simulink model "Andrej_Klein_zadanie2B"  (R2022b)
settings: Solver=VariableStepAuto  StartTime=0.0  StopTime=30  RelTol=1e-3
model workspace (MAT data in the model file):
  FSX1 : sugfis (value not decoded)
  FSX2 : sugfis (value not decoded)
  Sig = Simulink.Signal
  Sig.DataType = 'auto'
  Sig.Dimensions = -1
  Sig.DimensionsMode = 'auto'
  Sig.Complexity = 'auto'
  Sig.SampleTime = -1
  Sig.SamplingMode = 'auto'
  T = 0.1
  a0 = 14.3
  a1 = 10
  a2 = 28
  b1 = 13
libraries: fuzblock x2, simulink x1
settings Model: Creator=hwswi  LastModifiedBy=hwswi
settings DataIOCC: ReturnWorkspaceOutputs=off

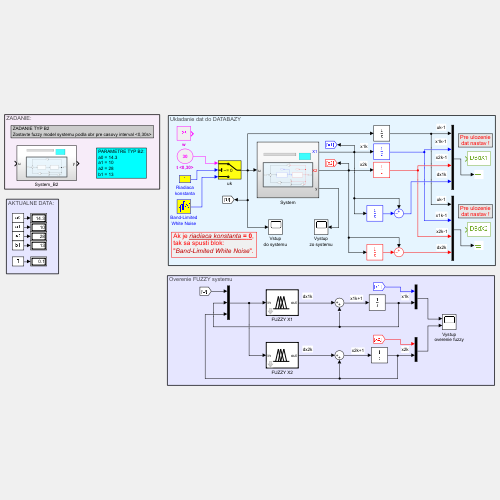
[thumbnail: Simulink's stored preview of the top-level diagram]
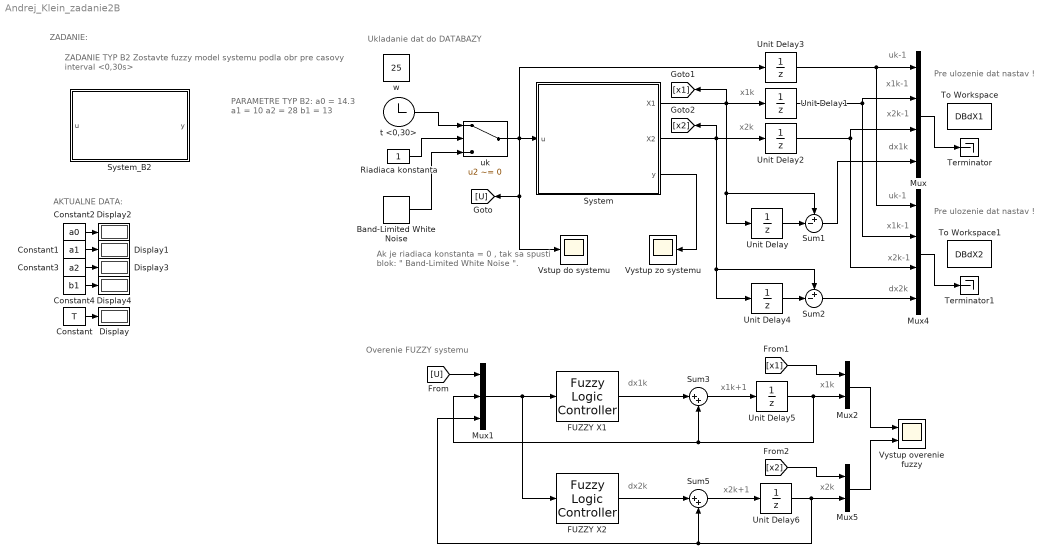
== system Andrej_Klein_zadanie2B ==
  note: Pre ulozenie
      | dat nastav !
  note: Ak je riadiaca konstanta = 0 ,
      | tak sa spusti blok:
      | " Band-Limited White Noise ".
  note: dx2k
  note: x1k+1
  note: x1k
  note: x1k
  note: uk-1
  note: Overenie FUZZY systemu
  note: AKTUALNE DATA:
  note: ZADANIE:
  note: Ukladanie dat do DATABAZY
  note: ZADANIE TYP B2
      | Zostavte fuzzy model systemu podla obr pre casovy interval <0,30s>
  note: PARAMETRE TYP B2:
      | a0 = 14.3
      | a1 = 10
      | a2 = 28
      | b1 = 13
  note: x1k-1
  note: dx1k
  note: x2k-1
  note: dx2k
  note: x2k
  note: x2k
  note: x2k+1
  note: dx1k
  note: uk-1
  note: x1k-1
  note: x2k-1
  note: Pre ulozenie
      | dat nastav !
  Band-Limited White Noise : simulink/Sources/Band-Limited White Noise  Cov=[500]  Ts=0.1  seed=[23341]
  Constant : Constant  Value=T
  Constant1 : Constant  Value=a1
  Constant2 : Constant  Value=a0
  Constant3 : Constant  Value=a2
  Constant4 : Constant  Value=b1
  Display{,1..4} (5 alike) : Display
  FUZZY X1 : fuzblock/Fuzzy Logic  Controller  FIS=FSX1  OutputSampleNumber=101  DataType=double  FuzzifiedInputs=off  RuleFiringStrengths=off  RuleOutputs=off  AggregatedOutputs=off  SimulateUsing=Interpreted execution  OutOfRangeInputValueMessage=warning  NoRuleFiredMessage=warning  EmptyOutputFuzzySetMessage=warning
  FUZZY X2 : fuzblock/Fuzzy Logic  Controller  FIS=FSX2  OutputSampleNumber=101  DataType=double  FuzzifiedInputs=off  RuleFiringStrengths=off  RuleOutputs=off  AggregatedOutputs=off  SimulateUsing=Interpreted execution  OutOfRangeInputValueMessage=warning  NoRuleFiredMessage=warning  EmptyOutputFuzzySetMessage=warning
  Mux : Mux
  Mux1 : Mux  Inputs=3
  Mux2 : Mux  Inputs=2
  Mux4 : Mux
  Mux5 : Mux  Inputs=2
  Riadiaca konstanta : Constant
  Sum1 : Sum  Inputs=+-|
  Sum2 : Sum  Inputs=+-|
  Sum3 : Sum  Inputs=|++
  Sum5 : Sum  Inputs=|++
  System : Subsystem
  System_B2 : Subsystem
  Terminator : Terminator
  Terminator1 : Terminator
  To Workspace : ToWorkspace  VariableName=DBdX1  SampleTime=0.1
  To Workspace1 : ToWorkspace  VariableName=DBdX2  SampleTime=0.1
  Unit Delay{,1..6} (7 alike) : UnitDelay  SampleTime=T
  Vstup do systemu : Scope
  Vystup overenie fuzzy : Scope  NumInputPorts=2
  Vystup zo systemu : Scope
  t <0,30> : Clock
  uk : Switch  Criteria=u2 ~= 0  Threshold=3  SaturateOnIntegerOverflow=off  InputSameDT=off
  w : Constant  Value=25
  wires:
  Constant/1 -> Display/1
  Constant1/1 -> Display1/1
  Constant2/1 -> Display2/1
  Constant3/1 -> Display3/1
  Constant4/1 -> Display4/1
  System/1(X1) -> [x1], Unit Delay1/1, Unit Delay/1, Sum1/1
  Unit Delay/1 -> Sum1/2
  Unit Delay4/1 -> Sum2/2
  System/2(X2) -> Unit Delay2/1, Sum2/1, Unit Delay4/1, [x2]
  Sum1/1 -> Mux/4
  Sum2/1 -> Mux4/4
  Unit Delay1/1 -> Mux/2, Mux4/2
  Unit Delay2/1 -> Mux4/3, Mux/3
  Unit Delay3/1 -> Mux/1, Mux4/1
  Sum3/1 -> Unit Delay5/1
  Unit Delay5/1 -> Sum3/2, Mux1/2, Mux2/2
  FUZZY X2/1 -> Sum5/1
  Unit Delay6/1 -> Mux5/2, Sum5/2, Mux1/3
  Sum5/1 -> Unit Delay6/1
  FUZZY X1/1 -> Sum3/1
  Mux5/1 -> Vystup overenie fuzzy/2
  Mux2/1 -> Vystup overenie fuzzy/1
  Mux1/1 -> FUZZY X2/1, FUZZY X1/1
  uk/1 -> System/1(u), [U], Vstup do systemu/1, Unit Delay3/1
  Riadiaca konstanta/1 -> uk/2
  Band-Limited White Noise/1 -> uk/3
  Mux/1 -> Terminator/1
  Mux4/1 -> Terminator1/1
  System/3(y) -> Vystup zo systemu/1
  [U] -> Mux1/1
  [x1] -> Mux2/1
  [x2] -> Mux5/1
  t <0,30>/1 -> uk/1

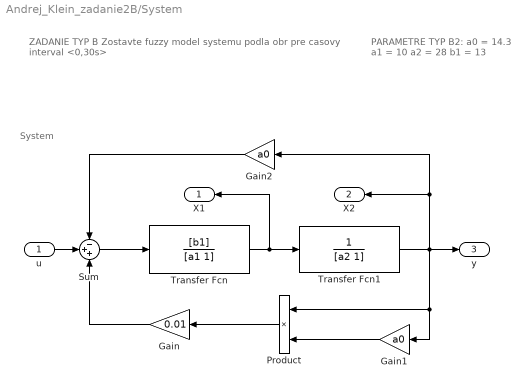
== system Andrej_Klein_zadanie2B/System ==
  note: System
  note: PARAMETRE TYP B2:
      | a0 = 14.3
      | a1 = 10
      | a2 = 28
      | b1 = 13
  note: ZADANIE TYP B
      | Zostavte fuzzy model systemu podla obr pre casovy interval <0,30s>
  u : Inport
  Gain : Gain  Gain=0.01
  Gain1 : Gain  Gain=a0
  Gain2 : Gain  Gain=a0
  Product : Product
  Sum : Sum  Inputs=-++
  Transfer Fcn : TransferFcn  Numerator=[b1]  Denominator=[a1 1]
  Transfer Fcn1 : TransferFcn  Denominator=[a2 1]
  X1 : Outport
  X2 : Outport  Port=2
  y : Outport  Port=3
  wires:
  Transfer Fcn/1 -> X1/1, Transfer Fcn1/1
  Transfer Fcn1/1 -> y/1, Gain2/1, X2/1, Gain1/1, Product/1
  Product/1 -> Gain/1
  Gain1/1 -> Product/2
  u/1 -> Sum/2
  Gain2/1 -> Sum/1
  Sum/1 -> Transfer Fcn/1
  Gain/1 -> Sum/3

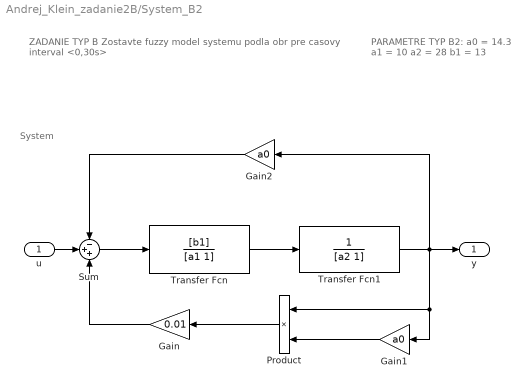
== system Andrej_Klein_zadanie2B/System_B2 ==
  note: System
  note: PARAMETRE TYP B2:
      | a0 = 14.3
      | a1 = 10
      | a2 = 28
      | b1 = 13
  note: ZADANIE TYP B
      | Zostavte fuzzy model systemu podla obr pre casovy interval <0,30s>
  u : Inport
  Gain : Gain  Gain=0.01
  Gain1 : Gain  Gain=a0
  Gain2 : Gain  Gain=a0
  Product : Product
  Sum : Sum  Inputs=-++
  Transfer Fcn : TransferFcn  Numerator=[b1]  Denominator=[a1 1]
  Transfer Fcn1 : TransferFcn  Denominator=[a2 1]
  y : Outport
  wires:
  Gain/1 -> Sum/3
  Transfer Fcn/1 -> Transfer Fcn1/1
  Gain2/1 -> Sum/1
  u/1 -> Sum/2
  Gain1/1 -> Product/2
  Product/1 -> Gain/1
  Sum/1 -> Transfer Fcn/1
  Transfer Fcn1/1 -> y/1, Gain2/1, Gain1/1, Product/1
